simulink model "testbench_mws"  (R2015a)
settings: Solver=ode3  StartTime=0.0  StopTime=inf  RelTol=1e-3
libraries: legoev3lib x8
settings Model: SimulationMode=external  CovModelRefEnable=off  ExtModeTrigDuration=2  Creator=Shobhit  LastModifiedBy=Shobhit
settings SolverCC: PositivePriorityOrder=on
settings DataIOCC: LimitDataPoints=off  SaveFormat=Dataset
settings OptimizationCC: OptimizeModelRefInitCode=on  LifeSpan=1  MaxStackSize=64
settings HardwareCC: ProdLargestAtomicInteger=Long  ProdLargestAtomicFloat=Float  ProdIntDivRoundTo=Zero  ProdEndianess=LittleEndian  ProdHWDeviceType=ARM Compatible->ARM 9
settings ModelReferenceCC: PropagateSignalLabelsOutOfModel=on
settings RTWCC: SystemTargetFile=ert.tlc  TLCOptions=-aInlineSetEventsForThisBaseRateFcn=TLC_FALSE -aSuppressMultiTaskScheduler=TLC_FALSE  TemplateMakefile=ert_default_tmf  Description=Embedded Coder  GenerateReport=on  Toolchain=Sourcery G++ Lite v2009q3  IncludeHyperlinkInReport=on  LaunchReport=on  GenerateTraceInfo=on  GenerateTraceReport=on  GenerateTraceReportSl=on  GenerateTraceReportSf=on  GenerateTraceReportEml=on
settings CodeAppCC: ForceParamTrailComments=on  IgnoreCustomStorageClasses=off  OperatorAnnotations=on  SimulinkDataObjDesc=on  SFDataObjDesc=on  MATLABFcnDesc=on  InsertBlockDesc=on  MATLABSourceComments=on
settings ERTTargetCC: GenerateSampleERTMain=off  ParMdlRefBuildCompliant=on  CompOptLevelCompliant=on  ConcurrentExecutionCompliant=on  ERTFirstTimeCompliant=on  SupportNonInlinedSFcns=on  ModelStepFunctionPrototypeControlCompliant=on  CPPClassGenCompliant=on  InlinedParameterPlacement=Hierarchical  ConvertIfToSwitch=on  SuppressUnreachableDefaultCases=on

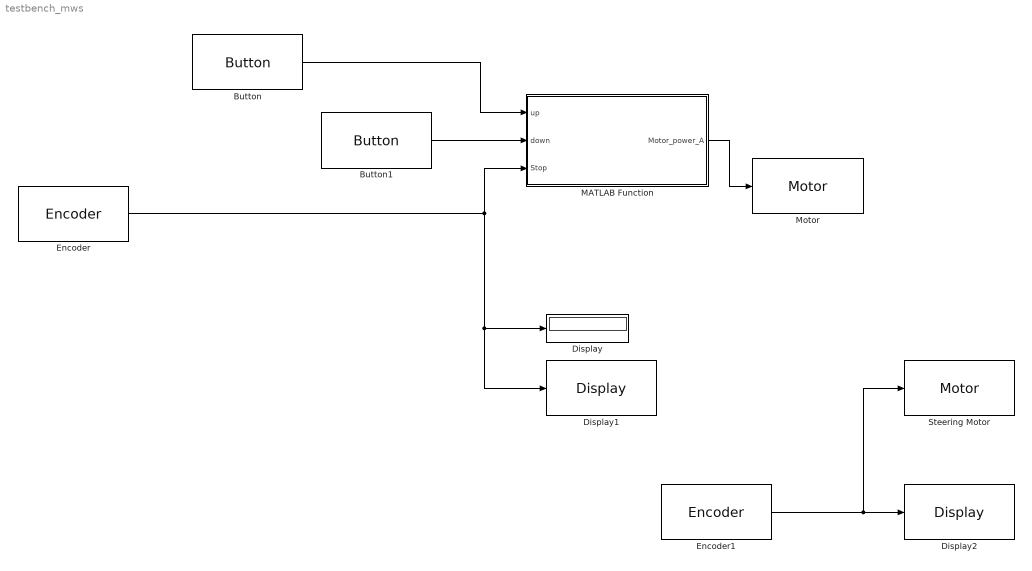
== system testbench_mws ==
  " Steering Motor" : legoev3lib/Motor  sportNumber=B  sstopAction=Brake
  Button : legoev3lib/Button  buttonType=Up  sampleTime=0.1
  Button1 : legoev3lib/Button  buttonType=Down  sampleTime=0.1
  Display : Display
      settings: Format=decimal (Stored Integer)
  Display1 : legoev3lib/Display  slcdStr=enc A  slcdLine=1  slcdFormat=Decimal
  Display2 : legoev3lib/Display  slcdStr=Enc B  slcdLine=2  slcdFormat=Decimal
  Encoder : legoev3lib/Encoder  portNumber=A  opMode=No reset  sampleTime=0.1
  Encoder1 : legoev3lib/Encoder  portNumber=B  opMode=Reset at each sample time  sampleTime=0.1
  MATLAB Function : MATLAB Function  TreatAsAtomicUnit=on
      settings: PermitHierarchicalResolution=ParametersOnly
  Motor : legoev3lib/Motor  sportNumber=A  sstopAction=Brake
  wires:
  Encoder1/1 -> " Steering Motor"/1, Display2/1
  MATLAB Function/1(Motor_power_A) -> Motor/1
  Encoder/1 -> MATLAB Function/3(Stop), Display1/1, Display/1
  Button/1 -> MATLAB Function/1(up)
  Button1/1 -> MATLAB Function/2(down)

== matlab function testbench_mws/MATLAB Function ==
  data: up input; down input; Motor_power_A output; Stop input
function Motor_power_A=fcn(up,down,Stop)
%#codegen
if(up==1)&&(Stop<=225)
    Motor_power_A=70;
elseif(down==1)&&(Stop>=-225)
    Motor_power_A=-70;
else
   Motor_power_A=0;
end
end
